simulink model "AAI_VVI"  (R2020a)
settings: Solver=FixedStepAuto  StartTime=0.0  StopTime=10.0  FixedStep=1e-3  RelTol=1e-3  EnableMultiTasking=on
settings Model: ExtModeTrigDuration=5  Creator=liams  LastModifiedBy=WinnieTrandinh
settings OptimizationCC: EnhancedBackFolding=on  PassReuseOutputArgsAs=Individual arguments  ZeroExternalMemoryAtStartup=off  ZeroInternalMemoryAtStartup=off  MaxStackSize=64  OptimizeBlockOrder=speed  DifferentSizesBufferReuse=on  OptimizationCustomize=off  EfficientTunableParamExpr=on
settings DebuggingCC: ParameterTunabilityLossMsg=error
settings HardwareCC: ProdBitPerPointer=32  ProdBitPerSizeT=32  ProdBitPerPtrDiffT=32  ProdLargestAtomicInteger=Long  ProdLargestAtomicFloat=Double  ProdWordSize=32  ProdHWDeviceType=ARM Compatible->ARM Cortex
settings SFSimCC: MATLABDynamicMemAlloc=off
settings RTWCC: SystemTargetFile=ert.tlc  HardwareBoard=NXP FRDM-K64F  TemplateMakefile=ert_default_tmf  Toolchain=GNU Tools for ARM Embedded Processors
settings CodeAppCC: ForceParamTrailComments=on  IgnoreCustomStorageClasses=off  OperatorAnnotations=on  SimulinkDataObjDesc=on  SFDataObjDesc=on  InsertBlockDesc=on

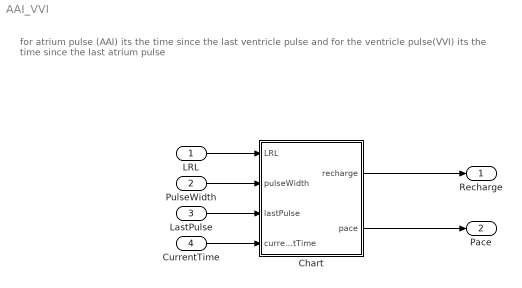
== system AAI_VVI ==
  note: for atrium pulse (AAI) its the time since the last ventricle pulse and for the ventricle pulse(VVI) its the time since the last atrium pulse
  LRL : Inport
  PulseWidth : Inport  Port=2
  LastPulse : Inport  Port=3
  CurrentTime : Inport  Port=4
  Chart : Stateflow chart  TreatAsAtomicUnit=on
  Recharge : Outport
  Pace : Outport  Port=2
  wires:
  Chart/2(pace) -> Pace/1
  Chart/1(recharge) -> Recharge/1
  LRL/1 -> Chart/1(LRL)
  LastPulse/1 -> Chart/3(lastPulse)
  CurrentTime/1 -> Chart/4(currentTime)
  PulseWidth/1 -> Chart/2(pulseWidth)

== stateflow chart AAI_VVI/Chart ==
  note: we will need it to pace if after a set delay the ventricle/atrium doesn't pump then the pacing will need to kick in
      | and pace for it
  state Pacing_Off
    entry:
    pace = false;
  state Recharge
    entry:
    recharge = true;
  note: t being the time since the last atrium/ventricle pulse
      | x being the time of the delay (x will need to be changed in the symbols panels because there is a
      | placeholder value there right now)
  note: update last pulse if inhibited
  state Pace
    entry:
    pace = true;
    recharge = false;
  (default) -> Pacing_Off
  Pacing_Off -> Recharge : [(currentTime-lastPulse)>LRL]
  Recharge -> Pace : [true]
  Pace -> Pacing_Off : [after(pulseWidth, msec)]
  data: recharge output; pace output; LRL input double =0.3; pulseWidth input; lastPulse input; currentTime input
